simulink model "esperimenti"  (R2022a)
settings: Solver=VariableStepAuto  StartTime=0.0  StopTime=100  RelTol=1e-3
values from neighbouring files (symbols this model uses):
  sys1 = tf(1,[10 1])    [esperimenti_sim.m]
  sys2 = tf(1,[100 1])    [esperimenti_sim.m]
settings Model: Creator=Stefano  LastModifiedBy=Stefano

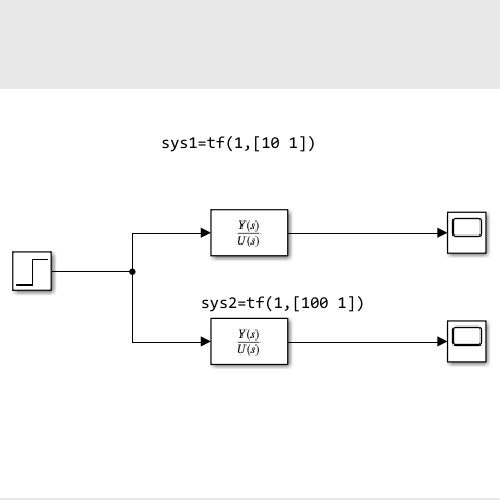
[thumbnail: Simulink's stored preview of the top-level diagram]
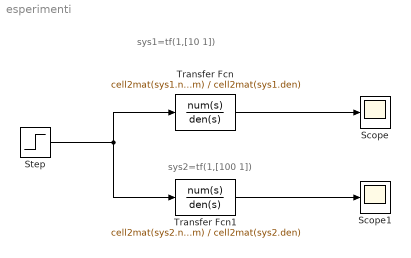
== system esperimenti ==
  note: sys2=tf(1,[100 1])
  note: sys1=tf(1,[10 1])
  Scope : Scope
  Scope1 : Scope
  Step : Step  SampleTime=0
  Transfer Fcn : TransferFcn  Numerator=cell2mat(sys1.num)  Denominator=cell2mat(sys1.den)
  Transfer Fcn1 : TransferFcn  Numerator=cell2mat(sys2.num)  Denominator=cell2mat(sys2.den)
  wires:
  Step/1 -> Transfer Fcn/1, Transfer Fcn1/1
  Transfer Fcn/1 -> Scope/1
  Transfer Fcn1/1 -> Scope1/1
